simulink model "massSpringDamper"  (R2023b)
settings: Solver=VariableStepAuto  StartTime=0.0  StopTime=20  RelTol=1e-3
undefined symbols (not defined in the file or in its folder): c, k, m
settings Model: Creator=Robin  LastModifiedBy=Robin

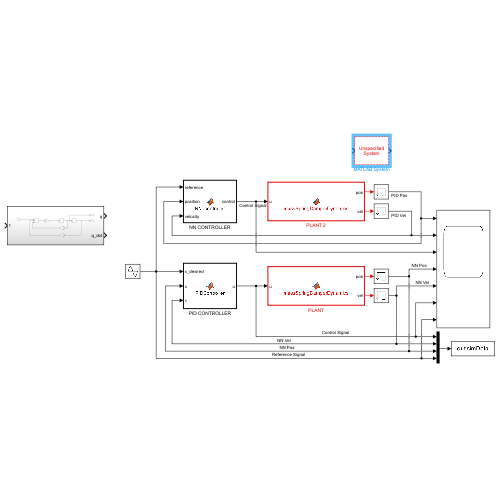
[thumbnail: Simulink's stored preview of the top-level diagram]
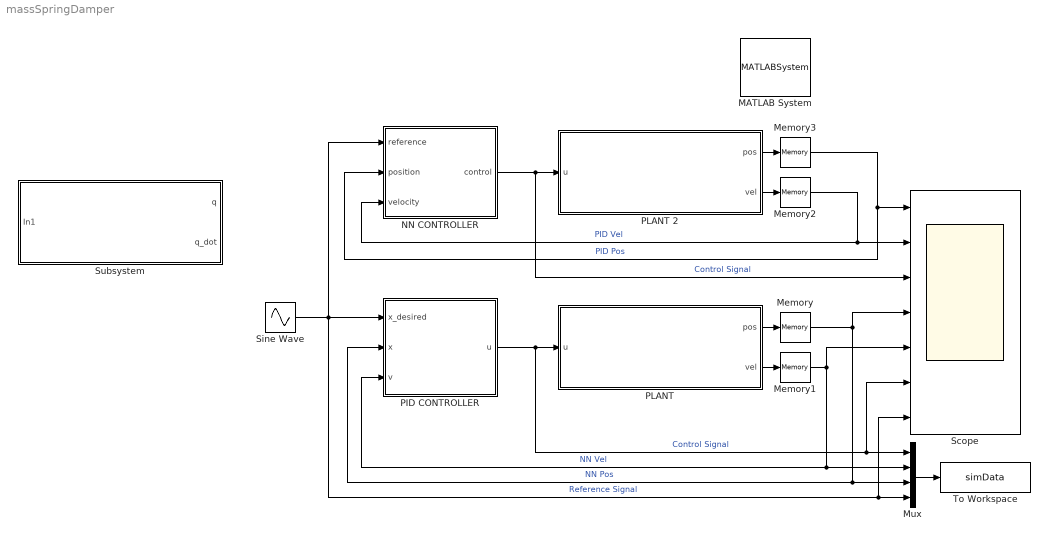
== system massSpringDamper ==
  MATLAB System : MATLABSystem
  Memory{,1..3} (4 alike) : Memory
  Mux : Mux
  NN CONTROLLER : MATLAB Function  TreatAsAtomicUnit=on
  PID CONTROLLER : MATLAB Function  TreatAsAtomicUnit=on
  PLANT : MATLAB Function  TreatAsAtomicUnit=on  SystemSampleTime=0.01
  PLANT 2 : MATLAB Function  TreatAsAtomicUnit=on  SystemSampleTime=0.01
  Scope : Scope  NumInputPorts=7
  Sine Wave : Sin  SampleTime=0
  Subsystem : Subsystem
  To Workspace : ToWorkspace  VariableName=simData  SaveFormat=Structure With Time  SampleTime=-1
  wires:
  Mux/1 -> To Workspace/1
  Sine Wave/1 -> PID CONTROLLER/1(x_desired), NN CONTROLLER/1(reference), Scope/7, Mux/4  "Reference Signal"
  PLANT/1(pos) -> Memory/1
  PLANT/2(vel) -> Memory1/1
  PID CONTROLLER/1(u) -> PLANT/1(u), Mux/1, Scope/6  "Control Signal"
  Memory/1 -> Scope/4, PID CONTROLLER/2(x), Mux/3  "NN Pos"
  Memory1/1 -> Scope/5, PID CONTROLLER/3(v), Mux/2  "NN Vel"
  PLANT 2/1(pos) -> Memory3/1
  PLANT 2/2(vel) -> Memory2/1
  Memory3/1 -> NN CONTROLLER/2(position), Scope/1  "PID Pos"
  Memory2/1 -> NN CONTROLLER/3(velocity), Scope/2  "PID Vel"
  NN CONTROLLER/1(control) -> Scope/3, PLANT 2/1(u)  "Control Signal"

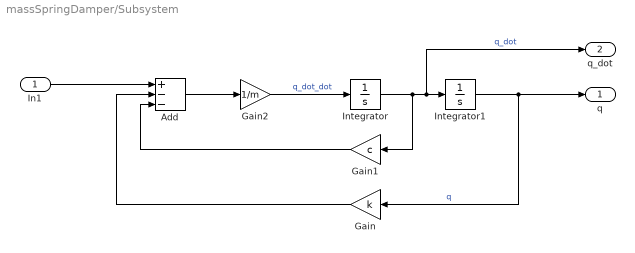
== system massSpringDamper/Subsystem ==
  In1 : Inport
  Add : Sum  Inputs=+--
  Gain : Gain  Gain=k
  Gain1 : Gain  Gain=c
  Gain2 : Gain  Gain=1/m
  Integrator : Integrator
  Integrator1 : Integrator
  q : Outport
  q_dot : Outport  Port=2
  wires:
  Gain/1 -> Add/2
  Gain2/1 -> Integrator/1  "q_dot_dot"
  Integrator1/1 -> q/1, Gain/1  "q"
  Gain1/1 -> Add/3
  Integrator/1 -> Gain1/1, q_dot/1, Integrator1/1  "q_dot"
  Add/1 -> Gain2/1
  In1/1 -> Add/1

== matlab function massSpringDamper/PID CONTROLLER ==
  settings: updateMethod=DISCRETE
  data: x_desired input; u output; x input; v input
function u = PIDController(x_desired, x, v)
% PIDController - Classic PID controller for mass-spring-damper system
%
% Inputs:
%   x_desired - Desired position (reference)
%   x         - Current position
%   v         - Current velocity
%
% Output:
%   u         - Control force

% Controller gains
Kp = 10;
Ki = 2;
Kd = 2;

% Sample time
Ts = 0.01;

% Persistent PID states
persistent integral_error prev_error
if isempty(integral_error)
    integral_error = 0;
    prev_error = 0;
end

% Compute errors
position_error = x_desired - x;
integral_error = integral_error + position_error * Ts;
derivative_error = (position_error - prev_error) / Ts;

% PID control law
u = Kp * position_error + Ki * integral_error + Kd * derivative_error;

% Optional: Saturation
% u = max(min(u, 10), -10);

% Update persistent state
prev_error = position_error;
end

== matlab function massSpringDamper/PLANT ==
  data: u input; pos output; vel output
function [pos, vel] = massSpringDamperDynamics(u)
% Discrete-time mass-spring-damper system
% u: input force (N)
% pos: output position (m)
% vel: output velocity (m/s)

% System parameters
m = 1.0;    % Mass (kg)
c = 0.5;    % Damping coefficient (Ns/m)
k = 2.0;    % Spring constant (N/m)
Ts = 0.01;  % Sample time (s)

% Persistent state variables
persistent x_prev v_prev
if isempty(x_prev)
    x_prev = 0; % Initial position
    v_prev = 0; % Initial velocity
end

% Compute acceleration
a = (u - c * v_prev - k * x_prev) / m;

% Update states using Euler integration
v = v_prev + Ts * a;
x = x_prev + Ts * v;

% Update persistent variables
v_prev = v;
x_prev = x;

% Output
pos = x;
vel = v;
end

== matlab function massSpringDamper/NN CONTROLLER ==
  data: reference input; control output; position input; velocity input
function control = NN_controller(reference, position, velocity)

input = [reference; position; velocity];

control = NNController(input);

== matlab function massSpringDamper/PLANT 2 ==
  data: u input; pos output; vel output
function [pos, vel] = massSpringDamperDynamics(u)
% Discrete-time mass-spring-damper system
% u: input force (N)
% pos: output position (m)
% vel: output velocity (m/s)

% System parameters
m = 1.0;    % Mass (kg)
c = 0.5;    % Damping coefficient (Ns/m)
k = 2.0;    % Spring constant (N/m)
Ts = 0.01;  % Sample time (s)

% Persistent state variables
persistent x_prev v_prev
if isempty(x_prev)
    x_prev = 0; % Initial position
    v_prev = 0; % Initial velocity
end

% Compute acceleration
a = (u - c * v_prev - k * x_prev) / m;

% Update states using Euler integration
v = v_prev + Ts * a;
x = x_prev + Ts * v;

% Update persistent variables
v_prev = v;
x_prev = x;

% Output
pos = x;
vel = v;
end
